simulink model "ZAD2_1_Model"  (R2018a)
settings: Solver=ode45  StartTime=0.0  StopTime=tend  MaxStep=Tp  RelTol=1e-3
values from neighbouring files (symbols this model uses):
  initConditionsAcc = [0 0]    [ZAD0_SRManCw2_Init.m]
  initConditionsVel = [0 0]    [ZAD0_SRManCw2_Init.m]
  Kp = diag([kp1, kp2])    [ZAD0_SRManCw2_Init.m]
  Kv = diag([kv1, kv2])    [ZAD0_SRManCw2_Init.m]
  omega1 = 0.1    [ZAD0_SRManCw2_Init.m]
  omega2 = 0.2    [ZAD0_SRManCw2_Init.m]
  Qd01 = 0.1    [ZAD0_SRManCw2_Init.m]
  Qd02 = 0.15    [ZAD0_SRManCw2_Init.m]
  Qd1 = 1.2    [ZAD0_SRManCw2_Init.m]
  Qd11 = 0.2    [ZAD0_SRManCw2_Init.m]
  Qd12 = 0.25    [ZAD0_SRManCw2_Init.m]
  Qd1const = 1.3    [ZAD0_SRManCw2_Init.m]
  Qd2 = 1.3    [ZAD0_SRManCw2_Init.m]
  Qd21 = 0.3    [ZAD0_SRManCw2_Init.m]
  Qd22 = 0.35    [ZAD0_SRManCw2_Init.m]
  Qd2const = 0.9    [ZAD0_SRManCw2_Init.m]
  Qd31 = 0.4    [ZAD0_SRManCw2_Init.m]
  Qd32 = 0.45    [ZAD0_SRManCw2_Init.m]
libraries: simulink x3
settings Model: Creator=szymon  LastModifiedBy=szymon

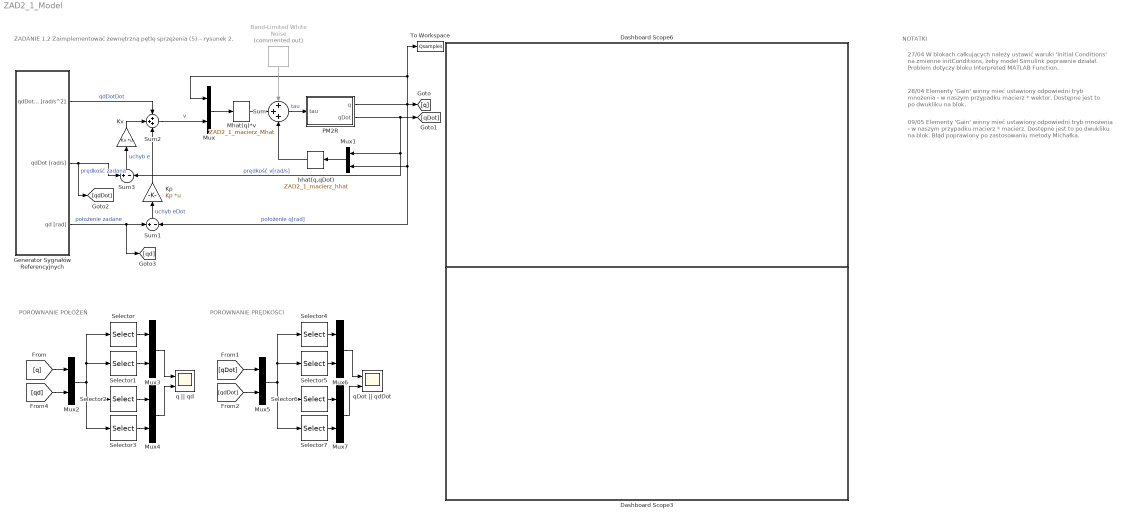
== system ZAD2_1_Model ==
  note: PORÓWNANIE POŁOŻEŃ
  note: NOTATKI
  note: ZADANIE 1.2
      |  Zaimplementować zewnętrzną pętlę sprzężenia (5) – rysunek 2.
  note: 27/04 W blokach całkujących należy ustawić waruki
      | 'Initial Conditions' na zmienne initConditions, żeby model
      | Simulink poprawnie działał. Problem dotyczy bloku
      | Interpreted MATLAB Function.
  note: 28/04 Elementy 'Gain' winny mieć ustawiony odpowiedni tryb
      | mnożenia - w naszym przypadku macierz * wektor.
      | Dostępne jest to po dwukliku na blok.
  note: PORÓWNANIE PRĘDKOŚCI
  note: 09/05 Elementy 'Gain' winny mieć ustawiony odpowiedni tryb
      | mnożenia - w naszym przypadku macierz * macierz.
      | Dostępne jest to po dwukliku na blok. Błąd poprawiony po
      | zastosowaniu metody Michałka.
  Band-Limited White Noise : simulink/Sources/Band-Limited White Noise  Commented=on  Cov=[0.1]  Ts=0.1  seed=[23341]
  Dashboard Scope3 : Subsystem  DialogController=hmiCreateDDGDialog  IsWebBlock=on  mask(MWDashboardBlock){webBlockId=7e31f546-b89a-4450-b53f-669fe20aafff, webBlockType=sdiscope, ShowInitialText=on, HMISrcModelName=ZAD2_1_Model}
      mask prompts: webBlockId "WebBlock Id"; webBlockType "WebBlock Type"; HMISrcModelName "Source Model"
      mask help: SimulinkHMI:dialogs:HMIScopeDialogDesc
      mask Help: helpview([docroot '/mapfiles/simulink.map'], 'hmi_scope')
      mask Display:
      | if strcmp(get_param(bdroot(gcb),'BlockDiagramType'), 'library')
      |     image([(matlabroot) '/toolbox/simulink/hmi/icons/DashboardScope.png']);
      | end
  Dashboard Scope6 : Subsystem  DialogController=hmiCreateDDGDialog  IsWebBlock=on  mask(MWDashboardBlock){webBlockId=060137c1-44cd-42f9-89eb-7b1da18c6d2d, webBlockType=sdiscope, ShowInitialText=on, HMISrcModelName=ZAD2_1_Model}
      mask prompts: webBlockId "WebBlock Id"; webBlockType "WebBlock Type"; HMISrcModelName "Source Model"
      mask help: SimulinkHMI:dialogs:HMIScopeDialogDesc
      mask Help: helpview([docroot '/mapfiles/simulink.map'], 'hmi_scope')
      mask Display:
      | if strcmp(get_param(bdroot(gcb),'BlockDiagramType'), 'library')
      |     image([(matlabroot) '/toolbox/simulink/hmi/icons/DashboardScope.png']);
      | end
  Generator Sygnałów Referencyjnych : Subsystem
  Kp : Gain  Gain=Kp  Multiplication=Matrix(K*u)
  Kv : Gain  Gain=Kv  Multiplication=Matrix(K*u)
  Mhat(q)*v : MATLABFcn  MATLABFcn=ZAD2_1_macierz_Mhat
  Mux{,1..7} (8 alike) : Mux  Inputs=2
  PM2R : Subsystem
  Selector : Selector  InputPortWidth=4  IndexOptions=Index vector (dialog)  Indices=[1]  OutputSizes=1
  Selector1 : Selector  InputPortWidth=4  IndexOptions=Index vector (dialog)  Indices=[3]  OutputSizes=1
  Selector2 : Selector  InputPortWidth=4  IndexOptions=Index vector (dialog)  Indices=[2]  OutputSizes=1
  Selector3 : Selector  InputPortWidth=4  IndexOptions=Index vector (dialog)  Indices=[4]  OutputSizes=1
  Selector4 : Selector  InputPortWidth=4  IndexOptions=Index vector (dialog)  Indices=[1]  OutputSizes=1
  Selector5 : Selector  InputPortWidth=4  IndexOptions=Index vector (dialog)  Indices=[3]  OutputSizes=1
  Selector6 : Selector  InputPortWidth=4  IndexOptions=Index vector (dialog)  Indices=[2]  OutputSizes=1
  Selector7 : Selector  InputPortWidth=4  IndexOptions=Index vector (dialog)  Indices=[4]  OutputSizes=1
  Sum : Sum  Inputs=+++
  Sum1 : Sum  Inputs=+-
  Sum2 : Sum  Inputs=+++
  Sum3 : Sum  Inputs=+-
  To Workspace : ToWorkspace  VariableName=Qsamples  SampleTime=-1
  hhat(q,qDot) : MATLABFcn  MATLABFcn=ZAD2_1_macierz_hhat
  q || qd : Scope  NumInputPorts=2
  qDot || qdDot : Scope  NumInputPorts=2
  wires:
  Mux/1 -> Mhat(q)*v/1
  Mux1/1 -> hhat(q,qDot)/1
  hhat(q,qDot)/1 -> Sum/3
  Mhat(q)*v/1 -> Sum/2
  Sum/1 -> PM2R/1(tau)  "tau"
  PM2R/2(qDot) -> [qDot], Mux1/1, Sum3/2  "prędkość v[rad/s]"
  Generator Sygnałów Referencyjnych/3(qd [rad]) -> [qd], Sum1/1  "położenie zadane"
  Sum1/1 -> Kp/1  "uchyb eDot"
  Sum2/1 -> Mux/2  "v"
  Generator Sygnałów Referencyjnych/1(qdDotDot [rad/s^2]) -> Sum2/1  "qdDotDot"
  Generator Sygnałów Referencyjnych/2(qdDot [rad/s]) -> [qdDot], Sum3/1  "prędkość zadana"
  Kv/1 -> Sum2/2
  Kp/1 -> Sum2/3
  Sum3/1 -> Kv/1  "uchyb e"
  PM2R/1(q) -> [q], Mux/1, To Workspace/1, Mux1/2, Sum1/2  "położenie q[rad]"
  Band-Limited White Noise/1 -> Sum/1
  [q] -> Mux2/1
  [qd] -> Mux2/2
  Selector/1 -> Mux3/1
  Selector1/1 -> Mux3/2
  Selector2/1 -> Mux4/1
  Selector3/1 -> Mux4/2
  Mux2/1 -> Selector3/1, Selector2/1, Selector1/1, Selector/1
  Mux3/1 -> q || qd/1
  Mux4/1 -> q || qd/2
  Selector6/1 -> Mux7/1
  Mux6/1 -> qDot || qdDot/1
  Mux7/1 -> qDot || qdDot/2
  Selector7/1 -> Mux7/2
  [qDot] -> Mux5/1
  Selector5/1 -> Mux6/2
  [qdDot] -> Mux5/2
  Selector4/1 -> Mux6/1
  Mux5/1 -> Selector7/1, Selector6/1, Selector5/1, Selector4/1

== system ZAD2_1_Model/Dashboard Scope3 ==

== system ZAD2_1_Model/Dashboard Scope6 ==

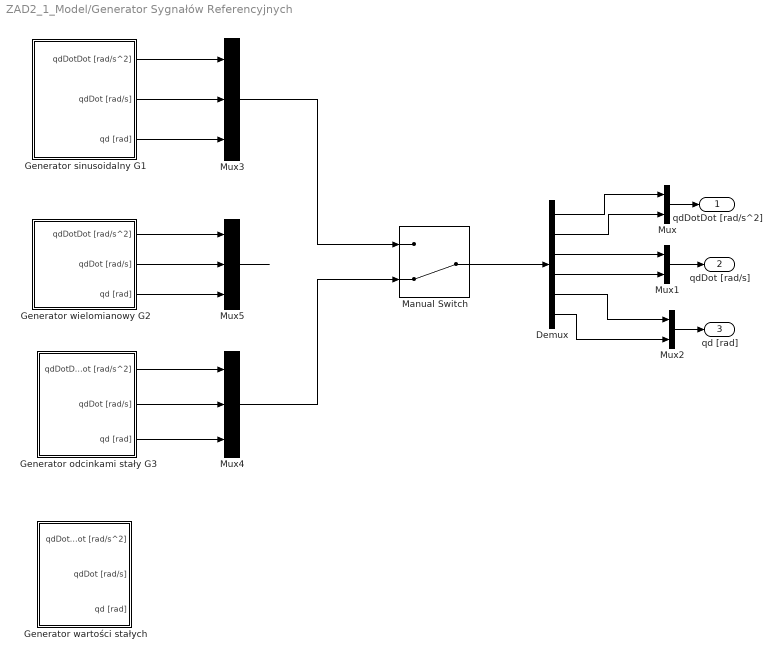
== system ZAD2_1_Model/Generator Sygnałów Referencyjnych ==
  Demux : Demux  Outputs=6
  "Generator odcinkami stały G3 " : Subsystem
  Generator sinusoidalny G1 : Subsystem
  Generator wielomianowy G2 : Subsystem
  Generator wartości stałych : Subsystem
  Manual Switch : ManualSwitch  CurrentSetting=0
  Mux : Mux  Inputs=2
  Mux1 : Mux  Inputs=2
  Mux2 : Mux  Inputs=2
  Mux3 : Mux  Inputs=3
  Mux4 : Mux  Inputs=3
  Mux5 : Mux  Inputs=3
  qdDotDot [rad/s^2] : Outport
  qdDot [rad/s] : Outport  Port=2
  qd [rad] : Outport  Port=3
  wires:
  Mux/1 -> qdDotDot [rad/s^2]/1
  Mux2/1 -> qd [rad]/1
  Mux1/1 -> qdDot [rad/s]/1
  Manual Switch/1 -> Demux/1
  Demux/1 -> Mux/1
  Demux/2 -> Mux/2
  Demux/3 -> Mux1/1
  Demux/4 -> Mux1/2
  Demux/5 -> Mux2/1
  Demux/6 -> Mux2/2
  Generator sinusoidalny G1/2(qdDot [rad/s]) -> Mux3/2
  Generator sinusoidalny G1/1(qdDotDot [rad/s^2]) -> Mux3/1
  Generator sinusoidalny G1/3(qd [rad]) -> Mux3/3
  Mux3/1 -> Manual Switch/1
  "Generator odcinkami stały G3 "/1(qdDotDot [rad/s^2]) -> Mux4/1
  "Generator odcinkami stały G3 "/2(qdDot [rad/s]) -> Mux4/2
  "Generator odcinkami stały G3 "/3(qd [rad]) -> Mux4/3
  Mux4/1 -> Manual Switch/2
  Generator wielomianowy G2/1(qdDotDot [rad/s^2]) -> Mux5/1
  Generator wielomianowy G2/2(qdDot [rad/s]) -> Mux5/2
  Generator wielomianowy G2/3(qd [rad]) -> Mux5/3
  Mux5/1 -> ?

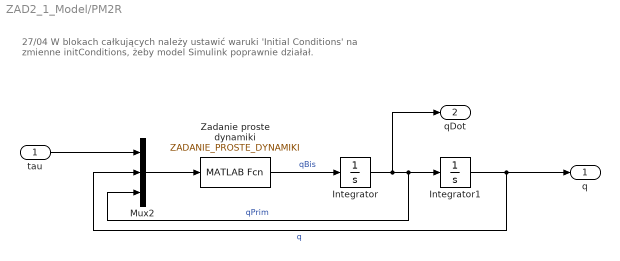
== system ZAD2_1_Model/PM2R ==
  note: 27/04 W blokach całkujących należy ustawić waruki 'Initial Conditions' na
      | zmienne initConditions, żeby model Simulink poprawnie działał.
  tau : Inport
  Integrator : Integrator  InitialCondition=initConditionsAcc
  Integrator1 : Integrator  InitialCondition=initConditionsVel
  Mux2 : Mux  Inputs=3
  Zadanie proste dynamiki : MATLABFcn  MATLABFcn=ZADANIE_PROSTE_DYNAMIKI
  q : Outport
  qDot : Outport  Port=2
  wires:
  Zadanie proste dynamiki/1 -> Integrator/1  "qBis"
  Integrator/1 -> qDot/1, Mux2/3, Integrator1/1  "qPrim"
  Integrator1/1 -> q/1, Mux2/2  "q"
  tau/1 -> Mux2/1
  Mux2/1 -> Zadanie proste dynamiki/1

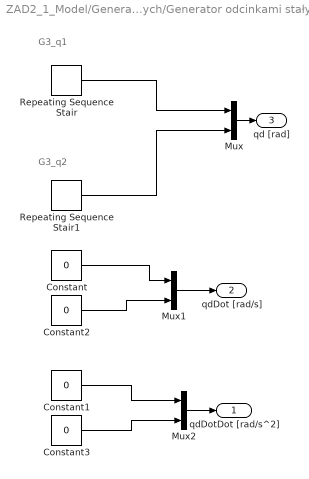
== system ZAD2_1_Model/Generator Sygnałów Referencyjnych/Generator odcinkami stały G3  ==
  note: G3_q2
  note: G3_q1
  Constant{,1..3} (4 alike) : Constant  Value=0
  Mux : Mux  Inputs=2
  Mux1 : Mux  Inputs=2
  Mux2 : Mux  Inputs=2
  Repeating Sequence Stair : simulink/Sources/Repeating Sequence Stair  OutValues=[Qd1const 0].'  tsamp=Ta  OutMin=[]  OutMax=[]  OutDataTypeStr=double  OutputDataTypeScalingMode=double  OutDataType=fixdt(0,8)  ConRadixGroup=Best Precision: Vector-wise  OutScaling=2^-12
  Repeating Sequence Stair1 : simulink/Sources/Repeating Sequence Stair  OutValues=[Qd2const 0].'  tsamp=Tb  OutMin=[]  OutMax=[]  OutDataTypeStr=double  OutputDataTypeScalingMode=double  OutDataType=fixdt(0,8)  ConRadixGroup=Best Precision: Vector-wise  OutScaling=2^-12
  qdDotDot [rad/s^2] : Outport
  qdDot [rad/s] : Outport  Port=2
  qd [rad] : Outport  Port=3
  wires:
  Constant/1 -> Mux1/1
  Repeating Sequence Stair1/1 -> Mux/2
  Repeating Sequence Stair/1 -> Mux/1
  Mux/1 -> qd [rad]/1
  Constant1/1 -> Mux2/1
  Constant2/1 -> Mux1/2
  Constant3/1 -> Mux2/2
  Mux2/1 -> qdDotDot [rad/s^2]/1
  Mux1/1 -> qdDot [rad/s]/1

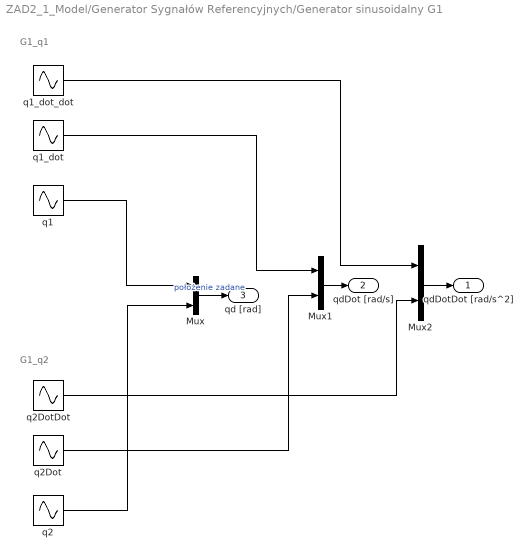
== system ZAD2_1_Model/Generator Sygnałów Referencyjnych/Generator sinusoidalny G1 ==
  note: G1_q2
  note: G1_q1
  Mux : Mux  Inputs=2
  Mux1 : Mux  Inputs=2
  Mux2 : Mux  Inputs=2
  "q1 " : Sin  Amplitude=Qd1  Frequency=omega1  SampleTime=0
  q1_dot : Sin  Amplitude=omega1*Qd1  Frequency=omega1  Phase=pi/2  SampleTime=0
  "q1_dot_dot " : Sin  Amplitude=-omega1^2*Qd1  Frequency=omega1  SampleTime=0
  q2 : Sin  Amplitude=Qd2  Frequency=omega2  SampleTime=0
  q2Dot : Sin  Amplitude=omega2*Qd2  Frequency=omega2  Phase=pi/2  SampleTime=0
  "q2DotDot " : Sin  Amplitude=-omega2^2*Qd2  Frequency=omega2  SampleTime=0
  qdDotDot [rad/s^2] : Outport
  qdDot [rad/s] : Outport  Port=2
  qd [rad] : Outport  Port=3
  wires:
  Mux1/1 -> qdDot [rad/s]/1
  Mux2/1 -> qdDotDot [rad/s^2]/1
  "q1_dot_dot "/1 -> Mux2/1
  "q2DotDot "/1 -> Mux2/2
  q2Dot/1 -> Mux1/2
  q1_dot/1 -> Mux1/1
  q2/1 -> Mux/2
  "q1 "/1 -> Mux/1
  Mux/1 -> qd [rad]/1  "położenie zadane"

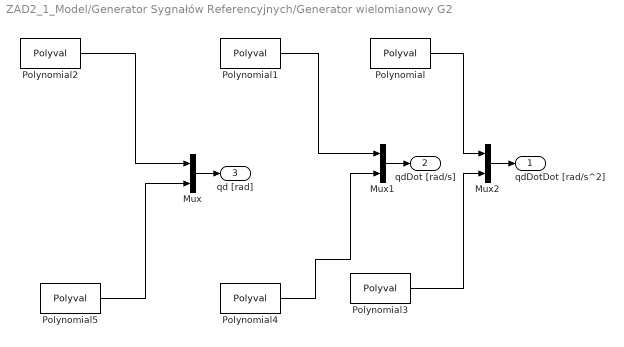
== system ZAD2_1_Model/Generator Sygnałów Referencyjnych/Generator wielomianowy G2 ==
  Mux : Mux  Inputs=2
  Mux1 : Mux  Inputs=2
  Mux2 : Mux  Inputs=2
  Polynomial : Polyval  Coefs=[6*Qd31*t, 2*Qd21]
  Polynomial1 : Polyval  Coefs=[3*Qd31*t.^2, 2*Qd21*t, Qd11]
  Polynomial2 : Polyval  Coefs=[Qd31*t.^3, Qd21*t.^2, Qd11*t, Qd01]
  Polynomial3 : Polyval  Coefs=[6*Qd32*t, 2*Qd22]
  Polynomial4 : Polyval  Coefs=[3*Qd32*t.^2, 2*Qd22*t, Qd12]
  Polynomial5 : Polyval  Coefs=[Qd32*t.^3, Qd22*t.^2, Qd12*t, Qd02]
  qdDotDot [rad/s^2] : Outport
  qdDot [rad/s] : Outport  Port=2
  qd [rad] : Outport  Port=3
  wires:
  Polynomial/1 -> Mux2/1
  Polynomial1/1 -> Mux1/1
  Polynomial2/1 -> Mux/1
  Polynomial3/1 -> Mux2/2
  Polynomial5/1 -> Mux/2
  Polynomial4/1 -> Mux1/2
  Mux/1 -> qd [rad]/1
  Mux1/1 -> qdDot [rad/s]/1
  Mux2/1 -> qdDotDot [rad/s^2]/1

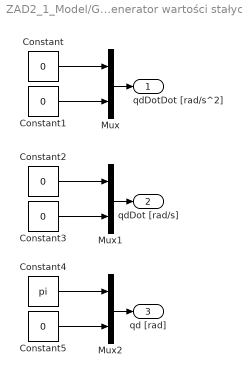
== system ZAD2_1_Model/Generator Sygnałów Referencyjnych/Generator wartości stałych ==
  Constant{,1..3,5} (5 alike) : Constant  Value=0
  Constant4 : Constant  Value=pi
  Mux : Mux  Inputs=2
  Mux1 : Mux  Inputs=2
  Mux2 : Mux  Inputs=2
  qdDotDot [rad/s^2] : Outport
  qdDot [rad/s] : Outport  Port=2
  qd [rad] : Outport  Port=3
  wires:
  Constant/1 -> Mux/1
  Mux/1 -> qdDotDot [rad/s^2]/1
  Constant1/1 -> Mux/2
  Constant2/1 -> Mux1/1
  Constant3/1 -> Mux1/2
  Mux1/1 -> qdDot [rad/s]/1
  Constant4/1 -> Mux2/1
  Constant5/1 -> Mux2/2
  Mux2/1 -> qd [rad]/1
